simulink model "prob49e_timevaryingmass"  (R2018a)
settings: Solver=ode4  StartTime=0.0  StopTime=300.0  FixedStep=0.001  RelTol=1e-3
values from neighbouring files (symbols this model uses):
  alfa = 3    [p49cConsts.m]
  beta = 5    [p49cConsts.m]
  k = 5    [p49cConsts.m]
  lambda_0 = 3    [p49cConsts.m]
  lambda_1 = 0.1    [p49cConsts.m]
  P0 = [3 0 0 ... (first row only)    [p49cConsts.m]
settings Model: Creator=Kristian  LastModifiedBy=Kristian
settings CodeAppCC: StateflowObjectComments=on

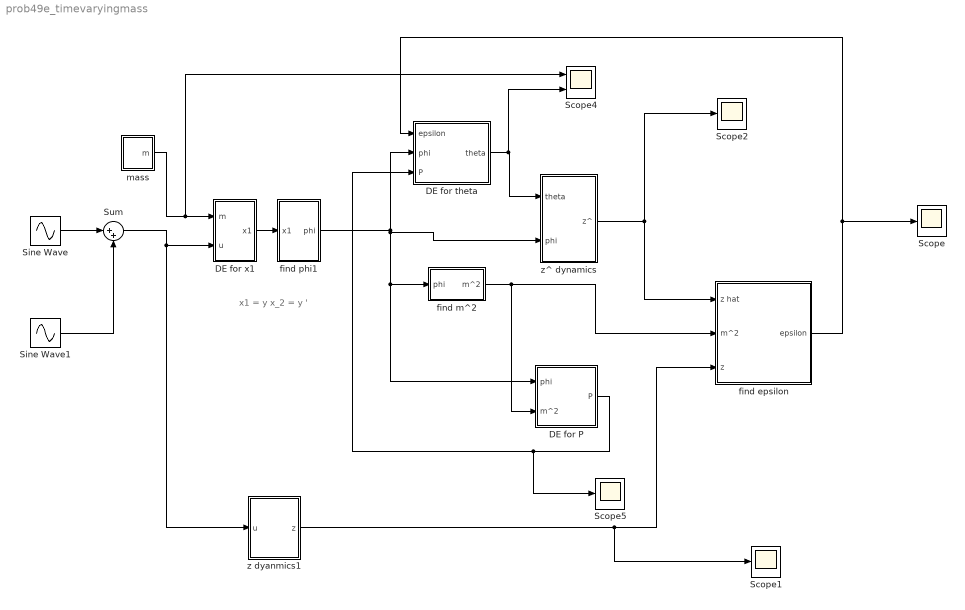
== system prob49e_timevaryingmass ==
  note: x1 = y
      | x_2 = y '
  DE for P : Subsystem
  DE for theta : Subsystem
  DE for x1 : Subsystem
  Scope{,1..2,5} (4 alike) : Scope
  Scope4 : Scope  NumInputPorts=2
  Sine Wave : Sin  Amplitude=5  Phase=0.3  SampleTime=0
  Sine Wave1 : Sin  Amplitude=7  Frequency=2  SampleTime=0
  Sum : Sum  Inputs=|++
  find epsilon : Subsystem
  find m^2 : Subsystem
  find phi1 : Subsystem
  "mass " : Subsystem
  z dyanmics1 : Subsystem
  z^ dynamics : Subsystem
  wires:
  find phi1/1("phi ") -> z^ dynamics/2(phi), DE for P/1("phi "), find m^2/1("phi "), DE for theta/2(phi)
  z^ dynamics/1("z^ ") -> Scope2/1, find epsilon/1(z hat)
  DE for theta/1("theta ") -> Scope4/2, z^ dynamics/1(theta)
  find epsilon/1("epsilon ") -> DE for theta/1("epsilon "), Scope/1
  z dyanmics1/1("z ") -> Scope1/1, find epsilon/3(z)
  find m^2/1("m^2 ") -> DE for P/2(m^2), find epsilon/2(m^2)
  DE for P/1("P ") -> Scope5/1, DE for theta/3(P)
  Sine Wave/1 -> Sum/1
  Sum/1 -> DE for x1/2(u), z dyanmics1/1(u)
  Sine Wave1/1 -> Sum/2
  "mass "/1(m) -> Scope4/1, DE for x1/1("m ")
  DE for x1/1("x1 ") -> find phi1/1(x1)

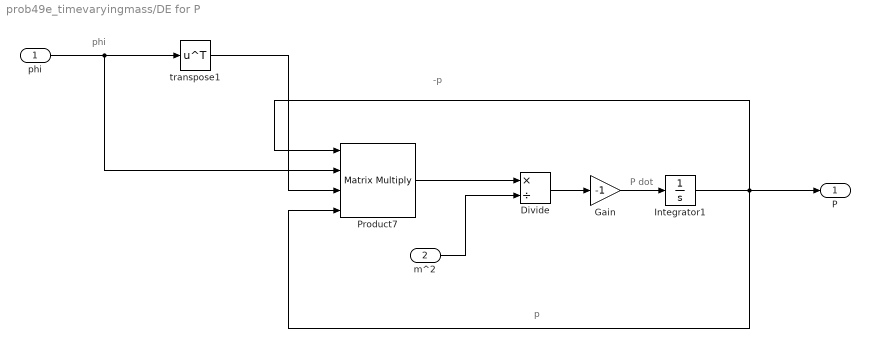
== system prob49e_timevaryingmass/DE for P ==
  note: P dot
  note: -p
  note: p
  note: phi
  "phi " : Inport
  m^2 : Inport  Port=2
  Divide : Product  Inputs=*/
  Gain : Gain  Gain=-1
  Integrator1 : Integrator  InitialCondition=P0
  Product7 : Product  Inputs=4  Multiplication=Matrix(*)
  transpose1 : Math  Operator=transpose  SaturateOnIntegerOverflow=on
  "P " : Outport
  wires:
  "phi "/1 -> Product7/2, transpose1/1
  transpose1/1 -> Product7/3
  Integrator1/1 -> Product7/4, Product7/1, "P "/1
  Product7/1 -> Divide/1
  m^2/1 -> Divide/2
  Divide/1 -> Gain/1
  Gain/1 -> Integrator1/1

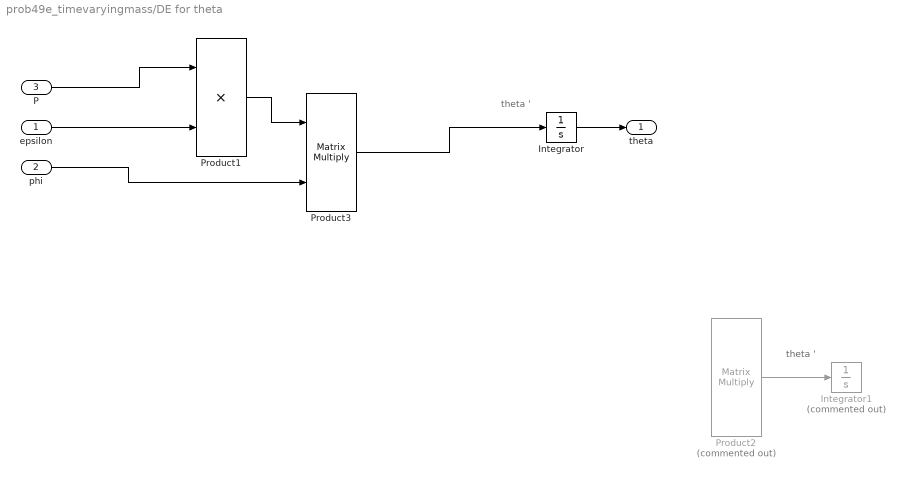
== system prob49e_timevaryingmass/DE for theta ==
  note: theta '
  note: theta '
  "epsilon " : Inport
  phi : Inport  Port=2
  P : Inport  Port=3
  Integrator : Integrator
  Integrator1 : Integrator  Commented=on
  Product1 : Product
  Product2 : Product  Commented=on  Inputs=3  Multiplication=Matrix(*)
  Product3 : Product  Multiplication=Matrix(*)
  "theta " : Outport
  wires:
  Integrator/1 -> "theta "/1
  P/1 -> Product1/1
  "epsilon "/1 -> Product1/2
  Product1/1 -> Product3/1
  phi/1 -> Product3/2
  Product3/1 -> Integrator/1
  Product2/1 -> Integrator1/1

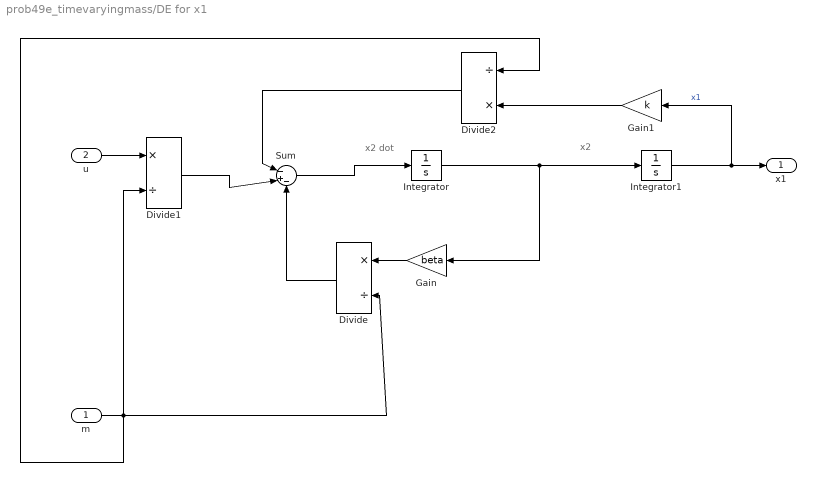
== system prob49e_timevaryingmass/DE for x1 ==
  note: x2 dot
  note: x2
  "m " : Inport
  u : Inport  Port=2
  Divide : Product  Inputs=*/
  Divide1 : Product  Inputs=*/
  Divide2 : Product  Inputs=/*
  Gain : Gain  Gain=beta
  Gain1 : Gain  Gain=k
  Integrator : Integrator
  Integrator1 : Integrator
  Sum : Sum  Inputs=|-+-
  "x1 " : Outport
  wires:
  Integrator/1 -> Integrator1/1, Gain/1
  Sum/1 -> Integrator/1
  Integrator1/1 -> Gain1/1, "x1 "/1  "x1"
  Gain/1 -> Divide/1
  "m "/1 -> Divide2/1, Divide/2, Divide1/2
  u/1 -> Divide1/1
  Gain1/1 -> Divide2/2
  Divide2/1 -> Sum/1
  Divide1/1 -> Sum/2
  Divide/1 -> Sum/3

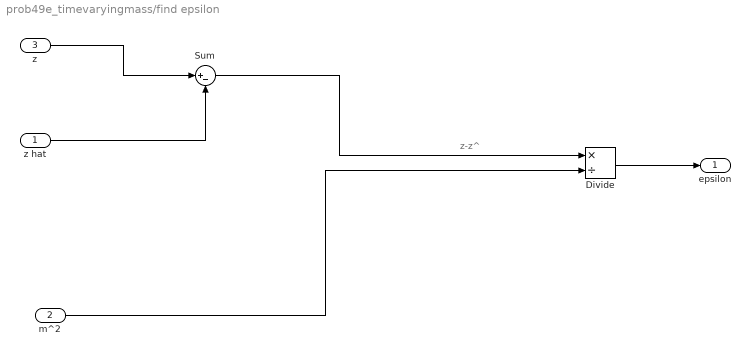
== system prob49e_timevaryingmass/find epsilon ==
  note: z-z^
  z hat : Inport
  m^2 : Inport  Port=2
  z : Inport  Port=3
  Divide : Product  Inputs=*/
  Sum : Sum  Inputs=|+-
  "epsilon " : Outport
  wires:
  z/1 -> Sum/1
  z hat/1 -> Sum/2
  m^2/1 -> Divide/2
  Sum/1 -> Divide/1
  Divide/1 -> "epsilon "/1

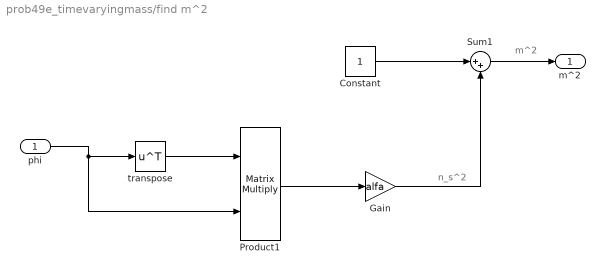
== system prob49e_timevaryingmass/find m^2 ==
  note: n_s^2
  note: m^2
  "phi " : Inport
  Constant : Constant
  Gain : Gain  Gain=alfa
  Product1 : Product  Multiplication=Matrix(*)
  Sum1 : Sum  Inputs=|++
  transpose : Math  Operator=transpose  SaturateOnIntegerOverflow=on
  "m^2 " : Outport
  wires:
  Constant/1 -> Sum1/1
  "phi "/1 -> Product1/2, transpose/1
  transpose/1 -> Product1/1
  Product1/1 -> Gain/1
  Gain/1 -> Sum1/2
  Sum1/1 -> "m^2 "/1

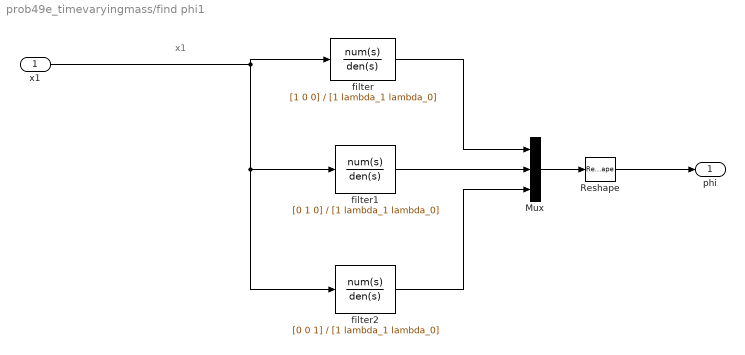
== system prob49e_timevaryingmass/find phi1 ==
  note: x1
  x1 : Inport
  Mux : Mux  Inputs=3
  Reshape : Reshape  OutputDimensionality=Column vector (2-D)
  filter : TransferFcn  Numerator=[1 0 0]  Denominator=[1 lambda_1 lambda_0]
  filter1 : TransferFcn  Numerator=[0 1 0]  Denominator=[1 lambda_1 lambda_0]
  filter2 : TransferFcn  Numerator=[0 0 1]  Denominator=[1 lambda_1 lambda_0]
  "phi " : Outport
  wires:
  x1/1 -> filter/1, filter2/1, filter1/1
  filter/1 -> Mux/1
  filter1/1 -> Mux/2
  filter2/1 -> Mux/3
  Mux/1 -> Reshape/1
  Reshape/1 -> "phi "/1

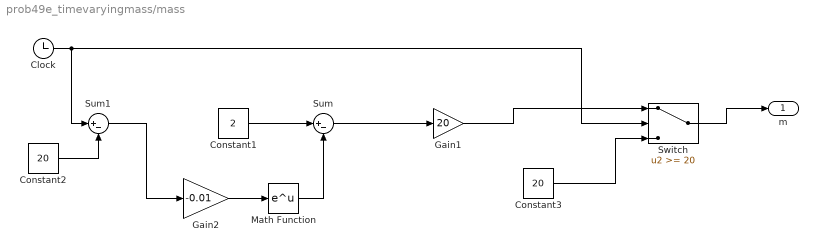
== system prob49e_timevaryingmass/mass  ==
  Clock : Clock
  Constant1 : Constant  Value=2
  Constant2 : Constant  Value=20
  Constant3 : Constant  Value=20
  Gain1 : Gain  Gain=20
  Gain2 : Gain  Gain=-0.01
  Math Function : Math  SaturateOnIntegerOverflow=on
  Sum : Sum  Inputs=|+-
  Sum1 : Sum  Inputs=|+-
  Switch : Switch  Threshold=20
  m : Outport
  wires:
  Clock/1 -> Sum1/1, Switch/2
  Switch/1 -> m/1
  Constant3/1 -> Switch/3
  Sum/1 -> Gain1/1
  Math Function/1 -> Sum/2
  Constant1/1 -> Sum/1
  Gain1/1 -> Switch/1
  Gain2/1 -> Math Function/1
  Constant2/1 -> Sum1/2
  Sum1/1 -> Gain2/1

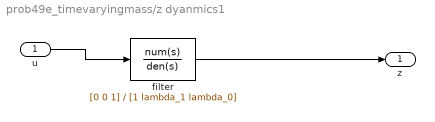
== system prob49e_timevaryingmass/z dyanmics1 ==
  u : Inport
  filter : TransferFcn  Numerator=[0 0 1]  Denominator=[1 lambda_1 lambda_0]
  "z " : Outport
  wires:
  u/1 -> filter/1
  filter/1 -> "z "/1

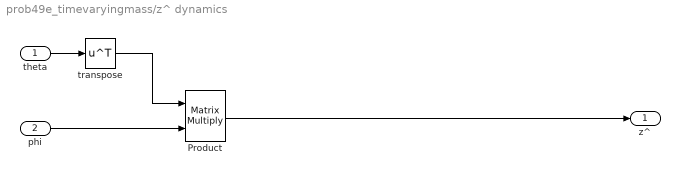
== system prob49e_timevaryingmass/z^ dynamics ==
  theta : Inport
  phi : Inport  Port=2
  Product : Product  Multiplication=Matrix(*)
  transpose : Math  Operator=transpose  SaturateOnIntegerOverflow=on
  "z^ " : Outport
  wires:
  Product/1 -> "z^ "/1
  theta/1 -> transpose/1
  transpose/1 -> Product/1
  phi/1 -> Product/2
